simulink model "model_1_Harness1"  (R2025a)
settings: Solver=FixedStepAuto  StartTime=0.0  StopTime=10.0  RelTol=1e-3
settings Model: Creator=z004f2se  LastModifiedBy=z004f2se

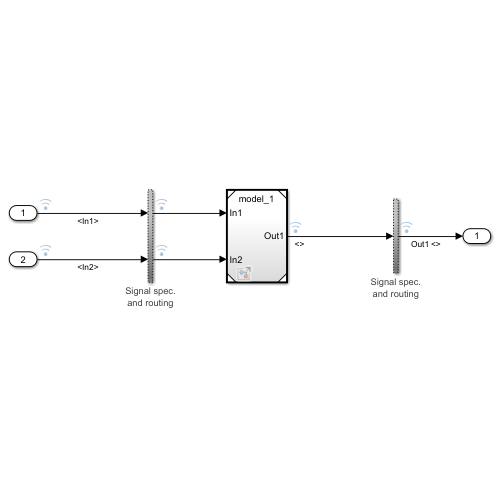
[thumbnail: Simulink's stored preview of the top-level diagram]
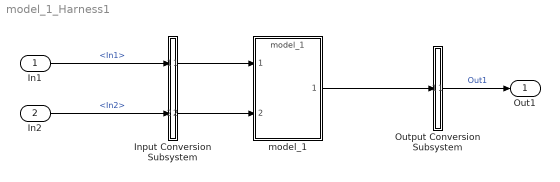
== system model_1_Harness1 ==
  In1 : Inport  OutDataTypeStr=double  PortDimensions=[1]  SampleTime=0.2
  In2 : Inport  Port=2  OutDataTypeStr=double  PortDimensions=[1]  SampleTime=0.2
  Input Conversion Subsystem : Subsystem  Tag=__SLT_ICS__  Description=|
      | Signal spec.
      | and routing
      settings: AttributesFormatString=%<Description>
  Output Conversion Subsystem : Subsystem  Tag=__SLT_OCS__  Description=|
      | Signal spec.
      | and routing
      settings: AttributesFormatString=%<Description>
  model_1 : ModelReference  ModelNameDialog=model_1  SimulationMode=Normal  ModelReferenceVersion=2.1
  Out1 : Outport
  wires:
  In1/1 -> Input Conversion Subsystem/1(Inport_1)  "<In1>"
  In2/1 -> Input Conversion Subsystem/2(Inport_2)  "<In2>"
  Output Conversion Subsystem/1(Outport_1) -> Out1/1  "Out1"
  Input Conversion Subsystem/1(Outport_1) -> model_1/1
  Input Conversion Subsystem/2(Outport_2) -> model_1/2
  model_1/1 -> Output Conversion Subsystem/1(Inport_1)

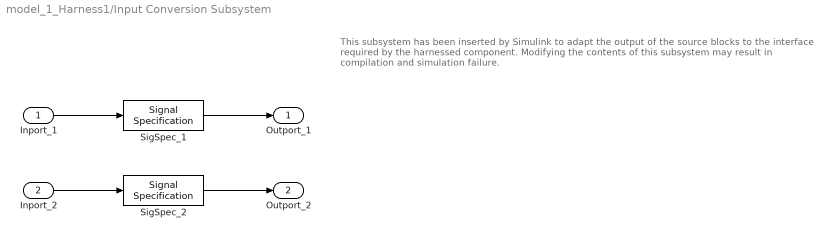
== system model_1_Harness1/Input Conversion Subsystem ==
  note: This subsystem has been inserted by Simulink to adapt the output of the source blocks to the interface required by the harnessed component.
      |  Modifying the contents of this subsystem may result in compilation and simulation failure.
  Inport_1 : Inport
  Inport_2 : Inport  Port=2
  SigSpec_1 : SignalSpecification  OutDataTypeStr=double  Dimensions=[1]  SampleTime=0.2
  SigSpec_2 : SignalSpecification  OutDataTypeStr=double  Dimensions=[1]  SampleTime=0.2
  Outport_1 : Outport
  Outport_2 : Outport  Port=2
  wires:
  SigSpec_1/1 -> Outport_1/1
  Inport_1/1 -> SigSpec_1/1
  SigSpec_2/1 -> Outport_2/1
  Inport_2/1 -> SigSpec_2/1

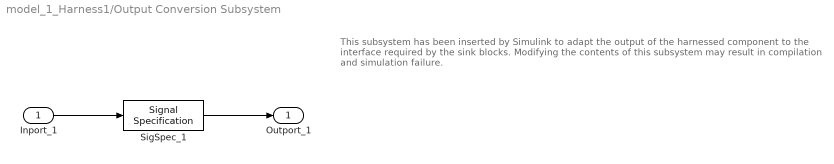
== system model_1_Harness1/Output Conversion Subsystem ==
  note: This subsystem has been inserted by Simulink to adapt the output of the harnessed component to the interface required by the sink blocks.
      |  Modifying the contents of this subsystem may result in compilation and simulation failure.
  Inport_1 : Inport
  SigSpec_1 : SignalSpecification  OutDataTypeStr=double  Dimensions=[1]  SampleTime=0.2
  Outport_1 : Outport
  wires:
  Inport_1/1 -> SigSpec_1/1
  SigSpec_1/1 -> Outport_1/1
